simulink model "mat3_PID_mega_V1"  (R2018a)
settings: Solver=FixedStepAuto  StartTime=0.0  StopTime=inf  RelTol=1e-3  EnableMultiTasking=on
libraries: arduinolib x4, simulink x2
settings Model: SimulationMode=external  ExtModeTrigDuration=2  Creator=MU  LastModifiedBy=MU
settings OptimizationCC: EnhancedBackFolding=on  PassReuseOutputArgsThreshold=0  MaxStackSize=64  OptimizeBlockOrder=speed  DifferentSizesBufferReuse=on  OptimizationCustomize=off
settings DebuggingCC: ParameterTunabilityLossMsg=error
settings HardwareCC: ProdBitPerInt=16  ProdBitPerPointer=16  ProdBitPerSizeT=16  ProdBitPerPtrDiffT=16  ProdLargestAtomicFloat=None  ProdWordSize=8  ProdHWDeviceType=Atmel->AVR  UseEmbeddedCoderFeatures=off  UseSimulinkCoderFeatures=off
settings SFSimCC: MATLABDynamicMemAlloc=off
settings RTWCC: SystemTargetFile=ert.tlc  HardwareBoard=Arduino Mega 2560  TLCOptions=-aInlineSetEventsForThisBaseRateFcn=TLC_FALSE -aSuppressMultiTaskScheduler=TLC_FALSE -aRateBasedStepFcn=1  TemplateMakefile=ert_default_tmf  GenerateReport=on  Toolchain=Arduino AVR  BuildConfiguration=Faster Runs  LaunchReport=on
settings CodeAppCC: ForceParamTrailComments=on  OperatorAnnotations=on  MangleLength=10
settings ERTTargetCC: ERTCustomFileBanners=off  SupportContinuousTime=on  SupportNonInlinedSFcns=on  RemoveResetFunc=off  SupportVariableSizeSignals=on  ModelStepFunctionPrototypeControlCompliant=off

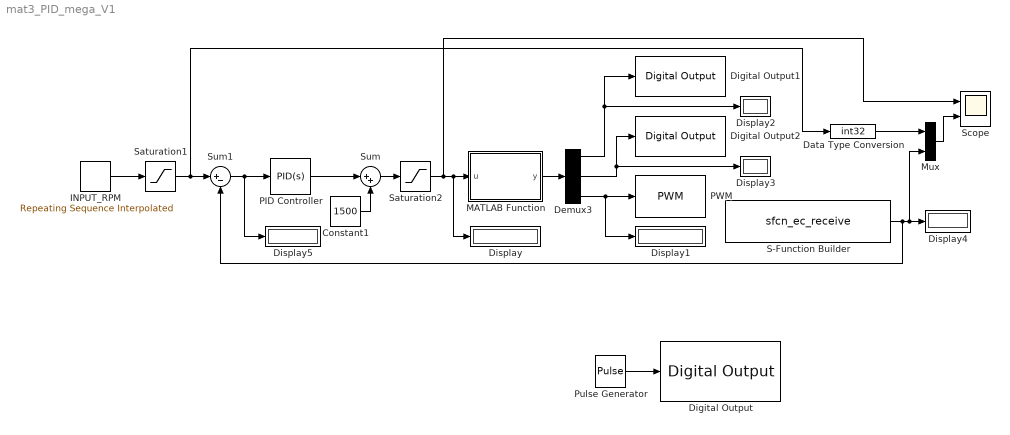
== system mat3_PID_mega_V1 ==
  Constant1 : Constant  Value=1500
  Data Type Conversion : DataTypeConversion  OutDataTypeStr=int32
  Demux3 : Demux  Outputs=3
  Digital Output : arduinolib/Digital Output  pinNumber=13  blockPlatform=arduino
  Digital Output1 : arduinolib/Digital Output  pinNumber=7  blockPlatform=arduino
  Digital Output2 : arduinolib/Digital Output  pinNumber=6  blockPlatform=arduino
  Display{,1..5} (6 alike) : Display
  INPUT_RPM : simulink/Sources/Repeating Sequence Interpolated  OutValues=[0 0 30000 30000 -30000 -30000 20000 5000 10000 0].'  TimeValues=[0 1 1.02 3 3.02 5 6 7 8 9].'  LookUpMeth=Interpolation-Use End Values  tsamp=0.02  OutMin=[]  OutMax=[]  OutDataTypeStr=double  OutputDataTypeScalingMode=double  OutDataType=fixdt(0,8)  OutScaling=2^-10
  MATLAB Function : MATLAB Function  TreatAsAtomicUnit=on
  Mux : Mux  Inputs=2
  PID Controller : simulink/Continuous/PID Controller  Controller=PID  TimeDomain=Continuous-time  SampleTime=-1  IntegratorMethod=Forward Euler  FilterMethod=Forward Euler  Form=Parallel  UseFilter=on  ControllerParametersSource=internal  P=10/1000  I=150/1000  D=0/1000  N=100  InitialConditionSource=internal  InitialConditionForIntegrator=0  InitialConditionForFilter=0  ExternalReset=none  LimitOutput=off  UpperSaturationLimit=inf  LowerSaturationLimit=-inf  LinearizeAsGain=on  AntiWindupMode=none  Kb=1  TrackingMode=off  Kt=1  PParamMin=[]  PParamMax=[]  IParamMin=[]  IParamMax=[]  DParamMin=[]  DParamMax=[]  NParamMin=[]  NParamMax=[]  KbParamMin=[]  KbParamMax=[]  KtParamMin=[]  KtParamMax=[]  POutMin=[]  POutMax=[]  IOutMin=[]  IOutMax=[]  DOutMin=[]  DOutMax=[]  NOutMin=[]  NOutMax=[]  KbOutMin=[]  KbOutMax=[]  KtOutMin=[]  KtOutMax=[]  IntegratorOutMin=[]  IntegratorOutMax=[]  FilterOutMin=[]  FilterOutMax=[]  SumOutMin=[]  SumOutMax=[]  SumI1OutMin=[]  SumI1OutMax=[]  SumI2OutMin=[]  SumI2OutMax=[]  SumI3OutMin=[]  SumI3OutMax=[]  SumDOutMin=[]  SumDOutMax=[]  SaturationOutMin=[]  SaturationOutMax=[]  IntegratorContinuousStateAttributes=''  IntegratorStateMustResolveToSignalObject=off  IntegratorRTWStateStorageClass=Auto  FilterContinuousStateAttributes=''  FilterStateMustResolveToSignalObject=off  FilterRTWStateStorageClass=Auto  DifferentiatorICPrevScaledInput=0  DifferentiatorOutMin=[]  DifferentiatorOutMax=[]  FilterDiffOutCoefMin=[]  FilterDiffOutCoefMax=[]  SumDenOutMin=[]  SumDenOutMax=[]  SumNumOutMin=[]  SumNumOutMax=[]  ReciprocalOutMin=[]  ReciprocalOutMax=[]  DivideOutMin=[]  DivideOutMax=[]  TunerSelectOption=Transfer Function Based (PID Tuner App)
  PWM : arduinolib/PWM  pinNumber=5  EnableInputFrequency=off  InitialFrequency=2000  InitialDutyCycle=0  NotificationType=None  blockPlatform=arduino
  Pulse Generator : DiscretePulseGenerator  PulseType=Time based  Period=0.5  PulseWidth=20
  S-Function Builder : S-Function  InitFcn=try, set_param(gcb,'FunctionName','sfcn_ec_receive'), end  FunctionName=sfcn_ec_receive  Parameters=uint8(2),uint8(3)  SFunctionModules=sfcn_ec_receive_wrapper  SFunctionDeploymentMode=off  EnableBusSupport=off  mask(S-Function Builder){}
      mask help: Simulink:masks:SFunctionBuilder_MD
      mask init:
      | val = [[.9  0.75 0.75 1 1 .9 .9 1]',[1 1 0.75 0.75 .9 .9 1 .9]'];try , sys = get_param(gcb,'SfunBuilderFcnName');if isempty(sys), sys = get_param(gcb,'FunctionName'); end,catch, sys = get_param(gcb,'FunctionName'); end
      settings: CopyFcn=set_param(gcbh,'LinkStatus','none')  PreSaveFcn=try, set_param(gcb,'FunctionName','sfcn_ec_receive'), end  OpenFcn=sfunctionwizard(gcbh)
      mask Display: plot(val(:,1),val(:,2)),disp(sys), port_label('output',1,'enc_rpm')
  Saturation1 : Saturate  UpperLimit=28000  LowerLimit=-28000
  Saturation2 : Saturate  UpperLimit=1850  LowerLimit=1150
  Scope : Scope  NumInputPorts=2
  Sum : Sum  Inputs=|++
  Sum1 : Sum  Inputs=|+-
  wires:
  MATLAB Function/1(y) -> Demux3/1
  Demux3/2 -> Display3/1, Digital Output2/1
  Demux3/3 -> Display1/1, PWM/1
  Demux3/1 -> Display2/1, Digital Output1/1
  Saturation2/1 -> Scope/1, Display/1, MATLAB Function/1(u)
  Pulse Generator/1 -> Digital Output/1
  S-Function Builder/1 -> Display4/1, Mux/2, Sum1/2
  Sum/1 -> Saturation2/1
  Sum1/1 -> PID Controller/1, Display5/1
  Saturation1/1 -> Data Type Conversion/1, Sum1/1
  Constant1/1 -> Sum/2
  Data Type Conversion/1 -> Mux/1
  Mux/1 -> Scope/2
  INPUT_RPM/1 -> Saturation1/1
  PID Controller/1 -> Sum/1

== matlab function mat3_PID_mega_V1/MATLAB Function ==
  data: u input; y output
function y = fcn(u)
if(u<700) %STOP
        INA1=0;
        INB1=0;
        PWM1=0;
elseif(u<1150) %CW, MAX SPEED
        INA1=1;
        INB1=0;
        PWM1=255;
elseif(u<1450) %CW, Speed control
        INA1=1;
        INB1=0;
        PWM1=(1450-u)/300*255;
elseif(u<1550) %STOP
        INA1=0;
        INB1=0;
        PWM1=0; %Free
        %PWM1=255; %Brake
elseif(u<1850) %CCW, Speed control
        INA1=0;
        INB1=1;
        PWM1=(u-1550)/300*255;
elseif(u<2300) %CCW, MAX SPEED
        INA1=0;
        INB1=1;
        PWM1=255;
else %STOP
        INA1=0;
        INB1=0;
        PWM1=0; 
end
y = [INA1;INB1;PWM1];
